simulink model "iiwa_IK_JT_ROS"  (R2016b)
settings: Solver=FixedStepAuto  StartTime=0.0  StopTime=inf  FixedStep=0.05  RelTol=1e-3
model workspace (MAT data in the model file):
  SL_ROS_VariableLengthArrays_MaxSizes.CommonInfo.ArrayTruncateAction = 'EmitWarning'
  SL_ROS_VariableLengthArrays_MaxSizes.MsgTypeMap = containers.Map
  SL_ROS_VariableLengthArrays_MaxSizes.MsgTypeMap.serialization.keys = {'sensor_msgs/JointState'}
  SL_ROS_VariableLengthArrays_MaxSizes.MsgTypeMap.serialization.values{1}(1).PropertyName = 'Name'
  SL_ROS_VariableLengthArrays_MaxSizes.MsgTypeMap.serialization.values{1}(1).DataType = 'std_msgs/String'
  SL_ROS_VariableLengthArrays_MaxSizes.MsgTypeMap.serialization.values{1}(1).MaxLength = 30
  SL_ROS_VariableLengthArrays_MaxSizes.MsgTypeMap.serialization.values{1}(2).PropertyName = 'Position'
  SL_ROS_VariableLengthArrays_MaxSizes.MsgTypeMap.serialization.values{1}(2).DataType = 'double'
  SL_ROS_VariableLengthArrays_MaxSizes.MsgTypeMap.serialization.values{1}(2).MaxLength = 128
  SL_ROS_VariableLengthArrays_MaxSizes.MsgTypeMap.serialization.values{1}(3).PropertyName = 'Velocity'
  SL_ROS_VariableLengthArrays_MaxSizes.MsgTypeMap.serialization.values{1}(3).DataType = 'double'
  SL_ROS_VariableLengthArrays_MaxSizes.MsgTypeMap.serialization.values{1}(3).MaxLength = 128
  SL_ROS_VariableLengthArrays_MaxSizes.MsgTypeMap.serialization.values{1}(4).PropertyName = 'Effort'
  SL_ROS_VariableLengthArrays_MaxSizes.MsgTypeMap.serialization.values{1}(4).DataType = 'double'
  SL_ROS_VariableLengthArrays_MaxSizes.MsgTypeMap.serialization.values{1}(4).MaxLength = 128
  SL_ROS_VariableLengthArrays_MaxSizes.MsgTypeMap.serialization.uniformity = 0
  SL_ROS_VariableLengthArrays_MaxSizes.MsgTypeMap.serialization.keyType = 'char'
  SL_ROS_VariableLengthArrays_MaxSizes.MsgTypeMap.serialization.valueType = 'any'
libraries: robotlib x5
(part 1 of 3)
settings Model: Creator=ram  LastModifiedBy=ram

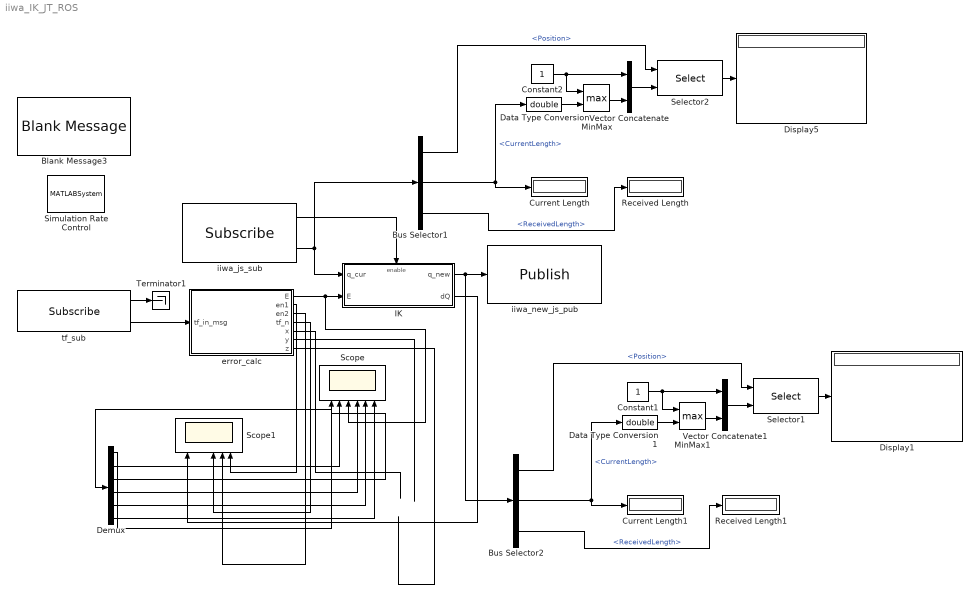
== system iiwa_IK_JT_ROS ==
  Blank Message3 : robotlib/Blank Message  SourceLibraryInfo=This block requires Robotics System Toolbox  messageType=tf2_msgs/TFMessage  SampleTime=inf
  Bus Selector1 : BusSelector  OutputSignals=Position,Position_SL_Info.CurrentLength,Position_SL_Info.ReceivedLength
  Bus Selector2 : BusSelector  OutputSignals=Position,Position_SL_Info.CurrentLength,Position_SL_Info.ReceivedLength
  Constant1 : Constant
  Constant2 : Constant
  Current Length : Display
  Current Length1 : Display
  Data Type Conversion : DataTypeConversion  OutDataTypeStr=double
  Data Type Conversion1 : DataTypeConversion  OutDataTypeStr=double
  Demux : Demux  Outputs=6
  Display1 : Display
  Display5 : Display
  IK : Subsystem
  MinMax : MinMax  Function=max  Inputs=2
  MinMax1 : MinMax  Function=max  Inputs=2
  Received Length : Display
  Received Length1 : Display
  Scope : Scope  NumInputPorts=6
  Scope1 : Scope  NumInputPorts=6
  Selector1 : Selector  IndexOptions=Starting and ending indices (port)  Indices=[2]  OutputSizes=1
  Selector2 : Selector  IndexOptions=Starting and ending indices (port)  Indices=[2]  OutputSizes=1
  Simulation Rate Control : MATLABSystem  System=ExampleHelperSimulationRateControl  SampleTime=0.05
      mask Type: ExampleHelperSimulationRateControl
      mask Display: disp('Rate Control');
  Terminator1 : Terminator
  Vector Concatenate : Concatenate
  Vector Concatenate1 : Concatenate
  error_calc : MATLAB Function  TreatAsAtomicUnit=on
  iiwa_js_sub : robotlib/Subscribe  SourceLibraryInfo=This block requires Robotics System Toolbox  topicSource=Select from ROS network  topic=/joint_states  messageType=sensor_msgs/JointState  sampleTime=-1  messageQueueLength=1
  iiwa_new_js_pub : robotlib/Publish  SourceLibraryInfo=This block requires Robotics System Toolbox  topicSource=Select from ROS network  topic=/arm_state  messageType=sensor_msgs/JointState  messageQueueLength=5
  tf_sub : robotlib/Subscribe  SourceLibraryInfo=This block requires Robotics System Toolbox  topicSource=Select from ROS network  topic=/tf  messageType=tf2_msgs/TFMessage  sampleTime=-1  messageQueueLength=1
  wires:
  tf_sub/2 -> error_calc/1(tf_in_msg)
  tf_sub/1 -> Terminator1/1
  iiwa_js_sub/1 -> IK/Enable
  error_calc/1(E) -> Demux/1, IK/2(E)
  iiwa_js_sub/2 -> Bus Selector1/1, IK/1(q_cur)
  Constant2/1 -> MinMax/1, Vector Concatenate/1
  Vector Concatenate/1 -> Selector2/2
  Bus Selector1/1 -> Selector2/1  "<Position>"
  Bus Selector1/2 -> Current Length/1, Data Type Conversion/1  "<CurrentLength>"
  Selector2/1 -> Display5/1
  Bus Selector1/3 -> Received Length/1  "<ReceivedLength>"
  MinMax/1 -> Vector Concatenate/2
  Data Type Conversion/1 -> MinMax/2
  error_calc/5(x) -> ?
  error_calc/6(y) -> ?
  error_calc/7(z) -> ?
  error_calc/2(en1) -> Scope1/6
  error_calc/3(en2) -> Scope1/5
  Demux/6 -> Scope/6
  Demux/5 -> Scope/5
  Demux/4 -> Scope/4
  Demux/3 -> Scope/3
  Demux/2 -> Scope/2
  Demux/1 -> Scope/1
  IK/2(dQ) -> Scope1/1
  error_calc/4(tf_n) -> Scope1/4
  IK/1(q_new) -> Bus Selector2/1, iiwa_new_js_pub/1
  Constant1/1 -> MinMax1/1, Vector Concatenate1/1
  Vector Concatenate1/1 -> Selector1/2
  Bus Selector2/1 -> Selector1/1  "<Position>"
  Bus Selector2/2 -> Current Length1/1, Data Type Conversion1/1  "<CurrentLength>"
  Selector1/1 -> Display1/1
  Bus Selector2/3 -> Received Length1/1  "<ReceivedLength>"
  MinMax1/1 -> Vector Concatenate1/2
  Data Type Conversion1/1 -> MinMax1/2

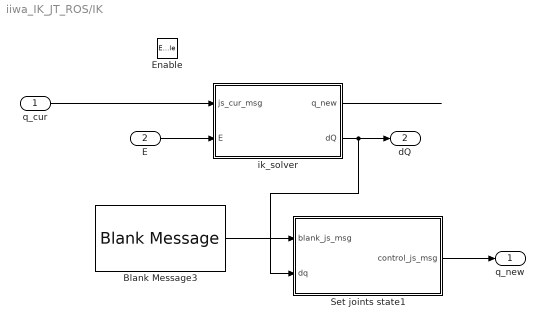
== system iiwa_IK_JT_ROS/IK ==
  q_cur : Inport
  E : Inport  Port=2
  Enable : EnablePort
  Blank Message3 : robotlib/Blank Message  SourceLibraryInfo=This block requires Robotics System Toolbox  messageType=sensor_msgs/JointState  SampleTime=inf
  Set joints state1 : MATLAB Function  TreatAsAtomicUnit=on
  ik_solver : MATLAB Function  TreatAsAtomicUnit=on
  q_new : Outport
  dQ : Outport  Port=2
  wires:
  ik_solver/1(q_new) -> ?
  E/1 -> ik_solver/2(E)
  q_cur/1 -> ik_solver/1(js_cur_msg)
  ik_solver/2(dQ) -> Set joints state1/2(dq), dQ/1
  Blank Message3/1 -> Set joints state1/1(blank_js_msg)
  Set joints state1/1(control_js_msg) -> q_new/1

== matlab function iiwa_IK_JT_ROS/IK/Set joints state1 ==
  data: blank_js_msg input; control_js_msg output Bus: SL_Bus_iiwa_IK_JT_ROS_sensor_msgs_JointState; dq input
function control_js_msg  = fcn(blank_js_msg, dq)

persistent seq;
if isempty(seq)
    seq = 0;
end

str_array_of_jnames = {'iiwa_j1', 'iiwa_j2', 'iiwa_j3', 'iiwa_j4', 'iiwa_j5', 'iiwa_j6', 'iiwa_j7'};
control_js_msg = blank_js_msg;

th_num = length(str_array_of_jnames);
control_js_msg.Name_SL_Info.CurrentLength = uint32(th_num);

%sec = 0.0;
%tf_nums = tf_msg_in.Transforms_SL_Info.CurrentLength;
%if (tf_nums > 1)
%    sec = tf_msg_in.Transforms(1).Header.Stamp.Sec;
%end

for idx=1:th_num
    str = str_array_of_jnames{idx};
    str_length = length(str);
    control_js_msg.Name(idx).Data(1:str_length) = uint8(str);
    control_js_msg.Name(idx).Data_SL_Info.CurrentLength = uint32(str_length);
end

control_js_msg.Position_SL_Info.CurrentLength = uint32(th_num);
control_js_msg.Position(1) = double(dq(1));
control_js_msg.Position(2) = double(dq(2));
control_js_msg.Position(3) = double(dq(3));
control_js_msg.Position(4) = double(dq(4));
control_js_msg.Position(5) = double(dq(5));
control_js_msg.Position(6) = double(dq(6));
control_js_msg.Position(7) = double(dq(7));


control_js_msg.Header.Seq = uint32(seq);
seq = seq + 1;
end
